simulink model "project_task_2"  (R2012b)
settings: Solver=ode5  StartTime=0.0  StopTime=8  FixedStep=0.01  RelTol=1e-3
undefined symbols (not defined in the file or in its folder): sigbuilder_block
(part 1 of 2)
settings Model: ExtModeTrigDuration=5000  Creator=adith  LastModifiedBy=adith
settings SolverCC: PositivePriorityOrder=on
settings RTWCC: SystemTargetFile=quarc_win64.tlc  TemplateMakefile=quarc_default_tmf  Description=QUARC Win64 Target  ProcessScript=quarc_win64_make_rtw_hook
settings STFCustomTargetCC: TargetPreCompLibLocation=C:\PROGRA~3\QUARC\lib\2012b\win64\release  CodeReplacementLibrary=ANSI_C  GeneratePreprocessorConditionals=Disable all  CombineOutputUpdateFcns=on  GRTInterface=off  SystemTargetFile=quarc_win64.tlc
settings GRTTargetCC: TargetPreCompLibLocation=C:\PROGRA~3\QUARC\lib\2012b\win64\release  ParMdlRefBuildCompliant=off  CompOptLevelCompliant=off  ConcurrentExecutionCompliant=off  MatFileLogging=off  ExtMode=on  ExtModeMexFile=quarc_comm

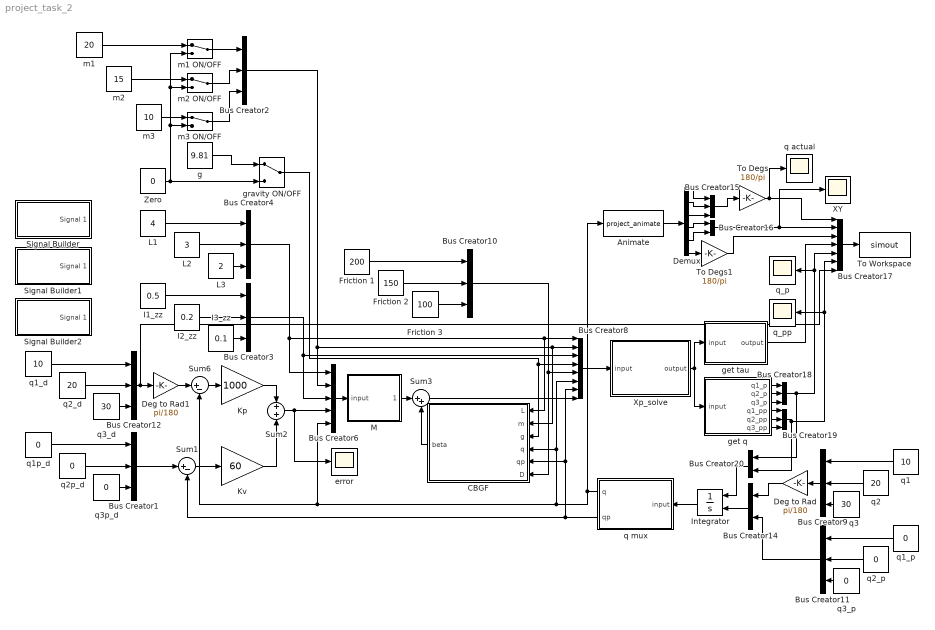
== system project_task_2 ==
  Animate : MATLABFcn  MATLABFcn=project_animate  OutputDimensions=6  OutputSignalType=real
  Bus Creator{1..4,9..12,15,18..19} (11 alike) : BusCreator  Inputs=3
  Bus Creator14 : BusCreator  Inputs=2
  Bus Creator16 : BusCreator  Inputs=2
  Bus Creator17 : BusCreator  Inputs=7
  Bus Creator20 : BusCreator  Inputs=2
  Bus Creator6 : BusCreator  Inputs=5
  Bus Creator8 : BusCreator  Inputs=8
  CBGF : MATLAB Function  TreatAsAtomicUnit=on
  Deg to Rad : Gain  Gain=pi/180
  Deg to Rad1 : Gain  Gain=pi/180
  Demux : Demux  Outputs=6
  Friction 1 : Constant  Value=200
  Friction 2 : Constant  Value=150
  Friction 3 : Constant  Value=100
  I1_zz : Constant  Value=0.5
  I2_zz : Constant  Value=0.2
  I3_zz : Constant  Value=0.1
  Integrator : Integrator  InitialConditionSource=external
  Kp : Gain  Gain=1000
  Kv : Gain  Gain=60
  L1 : Constant  Value=4
  L2 : Constant  Value=3
  L3 : Constant  Value=2
  M : MATLAB Function  TreatAsAtomicUnit=on
  Signal Builder : Subsystem  Tag=STV Subsys  LoadFcn=sigbuilder_block('load');  StartFcn=sigbuilder_block('start');  StopFcn=sigbuilder_block('stop');  ClipboardFcn=sigbuilder_block('clipboard');  mask(Sigbuilder block){}
      mask help: Simulink:masks:SigbuilderBlock_MD
      mask init:
      | if ~strcmp(get_param(bdroot(gcbh),'SimulationStatus'),'stopped') tuvar = sigbuilder_block('maskInit'); end
      settings: CopyFcn=sigbuilder_block('copy');  DeleteFcn=sigbuilder_block('delete');  ModelCloseFcn=sigbuilder_block('modelClose');  PreSaveFcn=sigbuilder_block('preSave');  PauseFcn=sigbuilder_block('pause');  ContinueFcn=sigbuilder_block('continue');  NameChangeFcn=sigbuilder_block('namechange');  OpenFcn=sigbuilder_block('open',[167.25 150.75 550.5 395.25 ]);  CloseFcn=sigbuilder_block('close');
      mask Display: plot(0, 0, 100, 100,[2, 2, 32, 32, 2], [68, 8, 8, 68, 68],[32, 2], [38, 38], [32, 19, 2],[53, 60, 44], [32, 17, 17, 2],[16, 16, 31, 31]);txt = getActiveGroup(gcbh);text(2, 100, txt,'verticalAlignment', 'top');
  Signal Builder1 : Subsystem  Tag=STV Subsys  LoadFcn=sigbuilder_block('load');  StartFcn=sigbuilder_block('start');  StopFcn=sigbuilder_block('stop');  ClipboardFcn=sigbuilder_block('clipboard');  mask(Sigbuilder block){}
      mask help: Simulink:masks:SigbuilderBlock_MD
      mask init:
      | if ~strcmp(get_param(bdroot(gcbh),'SimulationStatus'),'stopped') tuvar = sigbuilder_block('maskInit'); end
      settings: CopyFcn=sigbuilder_block('copy');  DeleteFcn=sigbuilder_block('delete');  ModelCloseFcn=sigbuilder_block('modelClose');  PreSaveFcn=sigbuilder_block('preSave');  PauseFcn=sigbuilder_block('pause');  ContinueFcn=sigbuilder_block('continue');  NameChangeFcn=sigbuilder_block('namechange');  OpenFcn=sigbuilder_block('open',[257.25 198 550.5 395.25 ]);  CloseFcn=sigbuilder_block('close');
      mask Display: plot(0, 0, 100, 100,[2, 2, 32, 32, 2], [68, 8, 8, 68, 68],[32, 2], [38, 38], [32, 19, 2],[53, 60, 44], [32, 17, 17, 2],[16, 16, 31, 31]);txt = getActiveGroup(gcbh);text(2, 100, txt,'verticalAlignment', 'top');
  Signal Builder2 : Subsystem  Tag=STV Subsys  LoadFcn=sigbuilder_block('load');  StartFcn=sigbuilder_block('start');  StopFcn=sigbuilder_block('stop');  ClipboardFcn=sigbuilder_block('clipboard');  mask(Sigbuilder block){}
      mask help: Simulink:masks:SigbuilderBlock_MD
      mask init:
      | if ~strcmp(get_param(bdroot(gcbh),'SimulationStatus'),'stopped') tuvar = sigbuilder_block('maskInit'); end
      settings: CopyFcn=sigbuilder_block('copy');  DeleteFcn=sigbuilder_block('delete');  ModelCloseFcn=sigbuilder_block('modelClose');  PreSaveFcn=sigbuilder_block('preSave');  PauseFcn=sigbuilder_block('pause');  ContinueFcn=sigbuilder_block('continue');  NameChangeFcn=sigbuilder_block('namechange');  OpenFcn=sigbuilder_block('open',[175.5 99 550.5 395.25 ]);  CloseFcn=sigbuilder_block('close');
      mask Display: plot(0, 0, 100, 100,[2, 2, 32, 32, 2], [68, 8, 8, 68, 68],[32, 2], [38, 38], [32, 19, 2],[53, 60, 44], [32, 17, 17, 2],[16, 16, 31, 31]);txt = getActiveGroup(gcbh);text(2, 100, txt,'verticalAlignment', 'top');
  Sum1 : Sum  Inputs=|+-
  Sum2 : Sum  Inputs=+|+
  Sum3 : Sum  Inputs=|++
  Sum6 : Sum  Inputs=|+-
  To Degs : Gain  Gain=180/pi
  To Degs1 : Gain  Gain=180/pi
  To Workspace : ToWorkspace  VariableName=simout  SampleTime=-1  SaveFormat=Structure With Time
  XY : Scope
      settings: ShowLegends=on  TimeRange=10  YMin=-8  YMax=9  SaveName=ScopeData4
  Xp_solve : MATLAB Function  TreatAsAtomicUnit=on
  Zero : Constant  Value=0
  error : Scope
      settings: ShowLegends=on  TimeRange=8  YMin=-2.75  YMax=2.5  SaveName=ScopeData3
  g : Constant  Value=9.81
  get q : MATLAB Function  TreatAsAtomicUnit=on
  get tau : MATLAB Function  TreatAsAtomicUnit=on
  gravity ON/OFF : ManualSwitch
  m1 : Constant  Value=20
  m1 ON/OFF : ManualSwitch
  m2 : Constant  Value=15
  m2 ON/OFF : ManualSwitch
  m3 : Constant  Value=10
  m3 ON/OFF : ManualSwitch
  q actual : Scope
      settings: ShowLegends=on  TimeRange=10  YMin=-100  YMax=175
  q mux : MATLAB Function  TreatAsAtomicUnit=on
  q1 : Constant  Value=10
  q1_d : Constant  Value=10
  q1_p : Constant  Value=0
  q1p_d : Constant  Value=0
  q2 : Constant  Value=20
  q2_d : Constant  Value=20
  q2_p : Constant  Value=0
  q2p_d : Constant  Value=0
  q3 : Constant  Value=30
  q3_d : Constant  Value=30
  q3_p : Constant  Value=0
  q3p_d : Constant  Value=0
  q_p : Scope
      settings: ShowLegends=on  TimeRange=20  YMin=-1.75  YMax=1.5
  q_pp : Scope
      settings: ShowLegends=on  TimeRange=20  YMin=-75  YMax=40  SaveName=ScopeData2
  wires:
  m1/1 -> m1 ON/OFF/1
  m3 ON/OFF/1 -> Bus Creator2/3
  m3/1 -> m3 ON/OFF/1
  m1 ON/OFF/1 -> Bus Creator2/1
  m2 ON/OFF/1 -> Bus Creator2/2
  m2/1 -> m2 ON/OFF/1
  Zero/1 -> m1 ON/OFF/2, m2 ON/OFF/2, m3 ON/OFF/2, gravity ON/OFF/2
  Friction 3/1 -> Bus Creator10/3
  Friction 2/1 -> Bus Creator10/2
  Friction 1/1 -> Bus Creator10/1
  g/1 -> gravity ON/OFF/1
  q1p_d/1 -> Bus Creator1/1
  q2p_d/1 -> Bus Creator1/2
  q3p_d/1 -> Bus Creator1/3
  I2_zz/1 -> Bus Creator3/2
  I3_zz/1 -> Bus Creator3/3
  L1/1 -> Bus Creator4/1
  L2/1 -> Bus Creator4/2
  L3/1 -> Bus Creator4/3
  Sum6/1 -> Kp/1
  Sum1/1 -> Kv/1
  Bus Creator1/1 -> Sum1/1
  Kp/1 -> Sum2/1
  Kv/1 -> Sum2/2
  Bus Creator4/1 -> CBGF/1(L), Bus Creator8/1, Bus Creator6/1
  Bus Creator2/1 -> CBGF/2(m), Bus Creator8/2, Bus Creator6/2
  Bus Creator3/1 -> Bus Creator6/3, Bus Creator8/3
  Sum2/1 -> error/1, Bus Creator6/4
  Bus Creator6/1 -> M/1(input)
  M/1(tau_wM) -> Sum3/1
  CBGF/1(beta) -> Sum3/2
  gravity ON/OFF/1 -> CBGF/3(g), Bus Creator8/4
  Bus Creator10/1 -> CBGF/6(D), Bus Creator8/5
  I1_zz/1 -> Bus Creator3/1
  Sum3/1 -> Bus Creator8/8
  Integrator/1 -> q mux/1(input)
  Bus Creator8/1 -> Xp_solve/1(input)
  q1/1 -> Bus Creator9/1
  q2/1 -> Bus Creator9/2
  q3/1 -> Bus Creator9/3
  q1_p/1 -> Bus Creator11/1
  q2_p/1 -> Bus Creator11/2
  q3_p/1 -> Bus Creator11/3
  Bus Creator11/1 -> Bus Creator14/2
  Bus Creator9/1 -> Deg to Rad/1
  Deg to Rad/1 -> Bus Creator14/1
  Bus Creator14/1 -> Integrator/2
  Bus Creator12/1 -> Bus Creator17/7, Deg to Rad1/1
  Deg to Rad1/1 -> Sum6/1
  q mux/1(q) -> Bus Creator8/6, CBGF/4(q), Bus Creator6/5, Sum6/2, Animate/1
  q mux/2(qp) -> Bus Creator8/7, CBGF/5(qp), Sum1/2
  Bus Creator17/1 -> To Workspace/1
  Animate/1 -> Demux/1
  Demux/1 -> Bus Creator15/1
  Demux/2 -> Bus Creator15/2
  Demux/3 -> Bus Creator15/3
  Bus Creator15/1 -> To Degs/1
  Demux/4 -> Bus Creator16/1
  Demux/5 -> Bus Creator16/2
  Demux/6 -> To Degs1/1
  To Degs/1 -> q actual/1, Bus Creator17/1
  Bus Creator16/1 -> XY/1, Bus Creator17/2
  To Degs1/1 -> Bus Creator17/3
  Xp_solve/1(output) -> get q/1(input), get tau/1(input)
  get tau/1(output) -> Bus Creator17/4
  Bus Creator18/1 -> Bus Creator20/1, q_p/1, Bus Creator17/5
  Bus Creator19/1 -> Bus Creator20/2, q_pp/1, Bus Creator17/6
  Bus Creator20/1 -> Integrator/1
  get q/1(q1_p) -> Bus Creator18/1
  get q/2(q2_p) -> Bus Creator18/2
  get q/3(q3_p) -> Bus Creator18/3
  get q/4(q1_pp) -> Bus Creator19/1
  get q/5(q2_pp) -> Bus Creator19/2
  get q/6(q3_pp) -> Bus Creator19/3
  q3_d/1 -> Bus Creator12/3
  q2_d/1 -> Bus Creator12/2
  q1_d/1 -> Bus Creator12/1

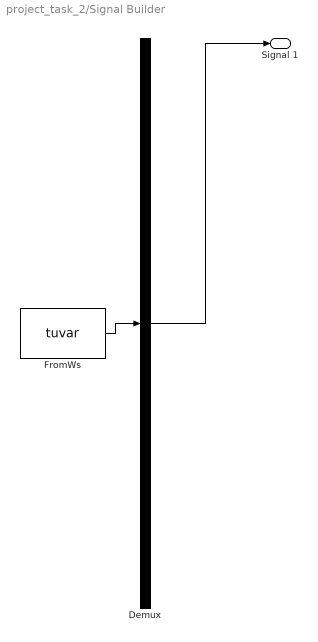
== system project_task_2/Signal Builder ==
  Demux : Demux  Tag=STV Demux  Outputs=1
  FromWs : FromWorkspace  Tag=STV FromWs  VariableName=tuvar  SampleTime=0
      SigBuilderData=|
      | common.afterFinalStr = 'Extrapolate'
      | common.sampleTime = 0
      | dataSet.timeRange = [0 10]
      | dataSet.name = 'Group 1'
      | sbobj.Groups.Name = 'Group 1'
      | sbobj.Groups.Signals.Name = 'Signal 1'
      | sbobj.Groups.Signals.XData = [0 0.5 0.5 4 6 10]
      | sbobj.Groups.Signals.YData = [10 10 -135 -135 -135 -135]
  Signal 1 : Outport  Tag=STV Outport
  wires:
  Demux/1 -> Signal 1/1
  FromWs/1 -> Demux/1

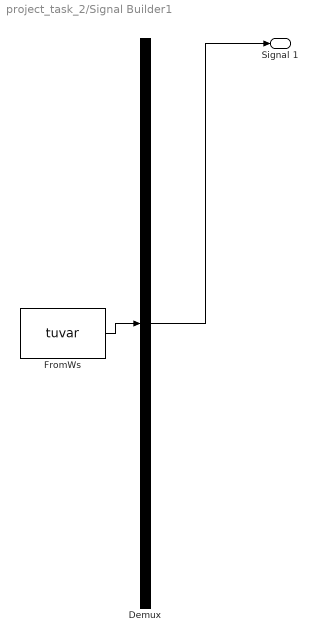
== system project_task_2/Signal Builder1 ==
  Demux : Demux  Tag=STV Demux  Outputs=1
  FromWs : FromWorkspace  Tag=STV FromWs  VariableName=tuvar  SampleTime=0
      SigBuilderData=|
      | common.afterFinalStr = 'Extrapolate'
      | common.sampleTime = 0
      | dataSet.timeRange = [0 10]
      | dataSet.name = 'Group 1'
      | sbobj.Groups.Name = 'Group 1'
      | sbobj.Groups.Signals.Name = 'Signal 1'
      | sbobj.Groups.Signals.XData = [0 3 3 6 10]
      | sbobj.Groups.Signals.YData = [20 20 150 150 150]
  Signal 1 : Outport  Tag=STV Outport
  wires:
  Demux/1 -> Signal 1/1
  FromWs/1 -> Demux/1

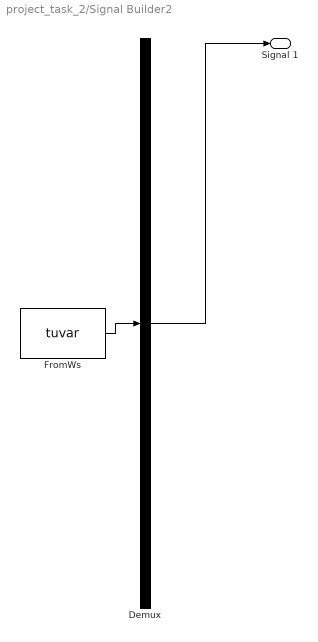
== system project_task_2/Signal Builder2 ==
  Demux : Demux  Tag=STV Demux  Outputs=1
  FromWs : FromWorkspace  Tag=STV FromWs  VariableName=tuvar  SampleTime=0
      SigBuilderData=|
      | common.afterFinalStr = 'Extrapolate'
      | common.sampleTime = 0
      | dataSet.timeRange = [0 10]
      | dataSet.name = 'Group 1'
      | sbobj.Groups.Name = 'Group 1'
      | sbobj.Groups.Signals.Name = 'Signal 1'
      | sbobj.Groups.Signals.XData = [0 5 5 6 10]
      | sbobj.Groups.Signals.YData = [30 30 -90 -90 -90]
  Signal 1 : Outport  Tag=STV Outport
  wires:
  Demux/1 -> Signal 1/1
  FromWs/1 -> Demux/1

== matlab function project_task_2/M ==
  data: input input; tau_wM output
function tau_wM  = M_matrix(input)
    L1 = input(1);
    L2 = input(2);
    L3 = input(3);
    m1 = input(4);
    m2 = input(5);
    m3 = input(6);
    I1_zz = input(7);
    I2_zz = input(8);
    I3_zz = input(9);
    tau1 = input(10);
    tau2 = input(11);
    tau3 = input(12);
    q1 = input(13);
    q2 = input(14);
    q3 = input(15);
%     g = input(10);
%     D1 = input(11);
%     D2 = input(12);
%     D3 = input(13);
    tau_p = [tau1; tau2; tau3];
    M = [(I1_zz + I2_zz + I3_zz + (L1^2*m1)/4 + L1^2*m2 + L1^2*m3 + (L2^2*m2)/4 + L2^2*m3 + (L3^2*m3)/4 + L1*L3*m3*cos(q2 + q3) + L1*L2*m2*cos(q2) + 2*L1*L2*m3*cos(q2) + L2*L3*m3*cos(q3)), (I2_zz + I3_zz + (L2^2*m2)/4 + L2^2*m3 + (L3^2*m3)/4 + (L1*L3*m3*cos(q2 + q3))/2 + (L1*L2*m2*cos(q2))/2 + L1*L2*m3*cos(q2) + L2*L3*m3*cos(q3)), (I3_zz + (L3^2*m3)/4 + (L1*L3*m3*cos(q2 + q3))/2 + (L2*L3*m3*cos(q3))/2);
         (I2_zz + I3_zz + (L2^2*m2)/4 + L2^2*m3 + (L3^2*m3)/4 + (L1*L3*m3*cos(q2 + q3))/2 + (L1*L2*m2*cos(q2))/2 + L1*L2*m3*cos(q2) + L2*L3*m3*cos(q3)),                                                                       (I2_zz + I3_zz + (L2^2*m2)/4 + L2^2*m3 + (L3^2*m3)/4 + L2*L3*m3*cos(q3)),                             ((m3*L3^2)/4 + (L2*m3*cos(q3)*L3)/2 + I3_zz);
         (I3_zz + (L3^2*m3)/4 + (L1*L3*m3*cos(q2 + q3))/2 + (L2*L3*m3*cos(q3))/2),                                                                                                   ((m3*L3^2)/4 + (L2*m3*cos(q3)*L3)/2 + I3_zz),                                                    ((m3*L3^2)/4 + I3_zz)];
    tau_wM = M*tau_p;
end

== matlab function project_task_2/CBGF ==
  data: L input; beta output; m input; g input; q input; qp input; D input
function beta  = CBGF(L, m, g, q, qp, D)
    L1 = L(1);
    L2 = L(2);
    L3 = L(3);
    m1 = m(1);
    m2 = m(2);
    m3 = m(3);
    q1 = q(1);
    q2 = q(2);
    q3 = q(3);
    q1_p = qp(1);
    q2_p = qp(2);
    q3_p = qp(3);
    D1 = D(1);
    D2 = D(2);
    D3 = D(3);
        
%     g = input(10);
%     D1 = input(11);
%     D2 = input(12);
%     D3 = input(13);

    G =[((5*g*(7*L2*cos(q1 + q2) + 14*L1*cos(q1) + 2*L3*cos(q1 + q2 + q3)))/2);
                  (5*L3*g*cos(q1 + q2 + q3) + (35*L2*g*cos(q1 + q2))/2);
                                             (5*L3*g*cos(q1 + q2 + q3))]; 
    F = [D1*q1_p;
        D2*q2_p;
        D3*q3_p];
    B = [ (-L1*(L3*m3*sin(q2 + q3) + L2*m2*sin(q2) + 2*L2*m3*sin(q2))), (-L3*m3*(L1*sin(q2 + q3) + L2*sin(q3))), (-L3*m3*(L1*sin(q2 + q3) + L2*sin(q3)));
                                                          0,                     (-L2*L3*m3*sin(q3)),                     (-L2*L3*m3*sin(q3));
                                           (L2*L3*m3*sin(q3)),                                     0,                                     0];

    C =[                                                             0, (-(L1*(L3*m3*sin(q2 + q3) + L2*m2*sin(q2) + 2*L2*m3*sin(q2)))/2), (-(L3*m3*(L1*sin(q2 + q3) + L2*sin(q3)))/2);
         ((L1*(L3*m3*sin(q2 + q3) + L2*m2*sin(q2) + 2*L2*m3*sin(q2)))/2),                                                              0,                     (-(L2*L3*m3*sin(q3))/2);
                              ((L3*m3*(L1*sin(q2 + q3) + L2*sin(q3)))/2),                                           ((L2*L3*m3*sin(q3))/2),                                         0];
    V =  C*[q1_p^2; q2_p^2; q3_p^2] + B*[q1_p*q2_p; q1_p*q3_p; q2_p*q3_p];
    beta = V + G + F;
end

== matlab function project_task_2/q mux ==
  data: input input; q output; qp output
function [q, qp]  = q_mux(input)
    q1 = input(1);
    q2 = input(2);
    q3 = input(3);
    q1_p = input(4);
    q2_p = input(5);
    q3_p = input(6);
    q = [q1, q2, q3];
    qp = [q1_p, q2_p, q3_p];
end

== matlab function project_task_2/get tau ==
  data: input input; output output
function output  = get_tau(input)
    tau1 = input(7);
    tau2 = input(8);
    tau3 = input(9);
    output = [tau1, tau2, tau3];
end

== matlab function project_task_2/get q ==
  data: input input; q1_p output; q2_p output; q3_p output; q1_pp output; q2_pp output; q3_pp output
function [q1_p, q2_p, q3_p, q1_pp, q2_pp, q3_pp]  = get_q(input)
    q1_p = input(1);
    q2_p = input(2);
    q3_p = input(3);
    q1_pp = input(4);
    q2_pp = input(5);
    q3_pp = input(6);
    %output = [q1_p, q2_p, q3_p, q1_pp, q2_pp, q3_pp];
end
